simulink model "AssembledTEST1"  (R2016b)
settings: Solver=VariableStepAuto  StartTime=0.0  StopTime=60  RelTol=1e-3
values from neighbouring files (symbols this model uses):
  ail_data = [ ... (first row only)    [lookup_init.m]
  Ap = pi * (D^2)/4    (= 5.69167367599)    [constants_init.m]
  Aw = 10.0    (= 10)    [constants_init.m]
  b = 15.85    [constants_init.m]
  beta0_data = [ ... (first row only)    [lookup_init.m]
  c0 = 2.3774    [constants_init.m]
  c_i = 1.847    [constants_init.m]
  cdrag_data = [ ... (first row only)    [lookup_init.m]
  clean_wing_data = [ ... (first row only)    [lookup_init.m]
  crt = 1.6764    [constants_init.m]
  CT_data = [ ... (first row only)    [lookup_init.m]
  D = 2.692    [constants_init.m]
  D0q_10 = 0.0778    [constants_init.m]
  D0q_20 = 0.2634    [constants_init.m]
  D0q_35 = 0.7099    [constants_init.m]
  DCDi_data = [ ... (first row only)    [lookup_init.m]
  DCM0b = -0.188    [constants_init.m]
  Deh_f_on_data = [ ... (first row only)    [lookup_init.m]
  Deh_on_data = [ ... (first row only)    [lookup_init.m]
  df = 1.981    [constants_init.m]
  DOWN_0 = HP * F2M    (= 1830.0192)    [InitialiseJ31.m]    (also in Trim.m = -xtrim(12))
  Dqhq_data = [ ... (first row only)    [lookup_init.m]
  e0 = d2r(2.0)    [constants_init.m]
  e_data10 = [ ... (first row only)    [lookup_init.m]
  e_data20 = [ ... (first row only)    [lookup_init.m]
  e_data35 = [ ... (first row only)    [lookup_init.m]
  EAST_0 = 0.0    (= 0)    [InitialiseJ31.m]    (also in Trim.m = xtrim(11))
  elaw_0 = -7.50225e+2    (= -750.225)    [constants_init.m]
  elaw_1 = 8.98698    [constants_init.m]
  elaw_2 = -6.94240e-3    (= -0.0069424)    [constants_init.m]
  FLAP = 0    [InitialiseJ31.m]
  flaps_lift_data = [ ... (first row only)    [lookup_init.m]
  flaps_moment_data = [ ... (first row only)    [lookup_init.m]
  flaps_tail_data = [ ... (first row only)    [lookup_init.m]
  flaps_wing_data = [ ... (first row only)    [lookup_init.m]
  fmc_data = [ ... (first row only)    [lookup_init.m]
  fmf_data = [ ... (first row only)    [lookup_init.m]
  fmn_data = [ ... (first row only)    [lookup_init.m]
  fus_data = [ ... (first row only)    [lookup_init.m]
  gamma_t = 0.578    [constants_init.m]
  h_data10 = [ ... (first row only)    [lookup_init.m]
  h_data20 = [ ... (first row only)    [lookup_init.m]
  h_data35 = [ ... (first row only)    [lookup_init.m]
  INERTIA = [IXX,IXY,IXZ;IXY,IYY,IYZ;IXZ,IYZ,IZZ]    [InitialiseJ31.m]
  it = d2r(-2.3)    [constants_init.m]
  iw = d2r(1.33)    [constants_init.m]
  Iwn2 = 0.636    [constants_init.m]
  J_W = 1.26    [constants_init.m]
  K1_data = [ ... (first row only)    [lookup_init.m]
  k1f_data = [ ... (first row only)    [lookup_init.m]
  k_data = [ ... (first row only)    [lookup_init.m]
  L_r0_10f = -0.0096    [constants_init.m]
  L_r0_20f = -0.0180    (= -0.018)    [constants_init.m]
  L_r0_35f = -0.0245    [constants_init.m]
  l_t = 11.6205 - 5.6642    (= 5.9563)    [constants_init.m]
  ld_data = [ ... (first row only)    [lookup_init.m]
  Lt = 4.686    [constants_init.m]
  Lt_dash = 247.1 * 0.3048/12    (= 6.27634)    [constants_init.m]
  Lv_b = -0.00145    [constants_init.m]
  Lv_h = 0.0445    [constants_init.m]
  Lv_n = 0.0165    [constants_init.m]
  mac = 1.716    [constants_init.m]
  mach_ffr = 0.4158    [constants_init.m]
  mach_pow = 0.7984    [constants_init.m]
  n = 1591/60    (= 26.5166666667)    [constants_init.m]
  NORTH_0 = 0.0    (= 0)    [InitialiseJ31.m]    (also in Trim.m = xtrim(10))
  Nr_b = -0.0060    (= -0.006)    [constants_init.m]
  Nv_n = -0.0005    [constants_init.m]
  Nv_wb = -0.0719    [constants_init.m]
  P_0 = 0.0    (= 0)    [InitialiseJ31.m]    (also in Trim.m = xtrim(4))
  pdrag_data = [ ... (first row only)    [lookup_init.m]
  PHI_0 = xtrim(7)    [Trim.m]
  piAt = At * pi    (= 17.5929188601)    [constants_init.m]
  piAw = Aw * pi    (= 31.4159265359)    [constants_init.m]
  PSI_0 = xtrim(9)    [Trim.m]
  Q_0 = 0.0    (= 0)    [InitialiseJ31.m]    (also in Trim.m = xtrim(5))
  R2D = 180/pi    (= 57.2957795131)    [InitialiseJ31.m]
  R_0 = 0.0    (= 0)    [InitialiseJ31.m]    (also in Trim.m = xtrim(6))
  s_e = 0.0954    [constants_init.m]
  side_data = [ ... (first row only)    [lookup_init.m]
  sideforce_data = [ ... (first row only)    [lookup_init.m]
  Sit = 1.874    [constants_init.m]
  Sn = 0.552    [constants_init.m]
  Sref = (pi/4) * df^2    (= 3.08218592191)    [constants_init.m]
  St = 7.785    [constants_init.m]
  Sw = 25.084    [constants_init.m]
  tail_data = [ ... (first row only)    [lookup_init.m]
  THETA_0 = xtrim(8)    [Trim.m]
  U_0 = xtrim(1)    [Trim.m]
  upwash_clean = [ ... (first row only)    [lookup_init.m]
  upwash_flaps = [ ... (first row only)    [lookup_init.m]
  V_0 = xtrim(2)    [Trim.m]
  vortex_drag_factors = [ ... (first row only)    [lookup_init.m]
  W_0 = xtrim(3)    [Trim.m]
  X_ci = ((223 - 140)*0.3048/12) - Xp_dash    (= 0.09144)    [constants_init.m]
  xacf = -6.653    [constants_init.m]
  xacn = (223 - 197.3)*0.3048/12    (= 0.65278)    [constants_init.m]
  xb0 = c0 * xb0_c0    (= 0.5895952)    [constants_init.m]
  xcit = -l_t - ycit * sin(d2r(11.31)) - (0.981/4)    [constants_init.m]
  Xp_dash = 79.4  * 0.3048/12    (= 2.01676)    [constants_init.m]
  xyz_p = [140.0*0.3048/12;-107.0*0.3048/12;11.5*0.3048/12]    [constants_init.m]
  xyz_s = [140.0*0.3048/12; 107.0*0.3048/12;11.5*0.3048/12]    [constants_init.m]
  ycit = 2.306    [constants_init.m]
  Yr_b = -0.0283    [constants_init.m]
  Yv_n = -0.0458    [constants_init.m]
  Yv_wb = -0.2627    [constants_init.m]
  Z_ht = 11.5*0.3048/12 - zact    (= 1.7271)    [constants_init.m]
  zacf = -1.741    [constants_init.m]
  zacn = 11.5*0.3048/12    (= 0.2921)    [constants_init.m]
  zact = -1.435    [constants_init.m]
  zacw = 0.929 - (3.307 * tan(d2r(7)))    [constants_init.m]
  Zt_dash = 12.0  * 0.3048/12    (= 0.3048)    [constants_init.m]
undefined symbols (not defined in the file or in its folder): CG, MASS
libraries: aerolibasang x3, aerolibatmos2 x1
(part 5 of 5)

== system AssembledTEST1/Subsystem/Powerplants and Slipstream/Subsystem2/Powerplant - starboard (forces and moments about spinner) (in body axes)/Propeller - right (forces and moments about spinner) (in body axes)/upwash at spinner ==
  In4 : Inport
  In1 : Inport  Port=2
  In3 : Inport  Port=3
  In2 : Inport  Port=4
  Add : Sum
  Constant : Constant
  Get_af : Sum
  Get_an : Sum  Inputs=+++
  Get_efi : Product  RndMeth=Zero
  Get_efo : Product  RndMeth=Zero
  Get_efw : Subsystem
      mask Display:
      | port_label('output',1,'\epsilon^f_{w}','texmode','on')
      | port_label('input',1,'flap')
      | port_label('input',2,'Mach')
      | port_label('input',3,'C_L','texmode','on')
  Get_ei : Sum  Inputs=+++
  Get_en : Product  RndMeth=Zero
  Get_enf : Product  RndMeth=Zero
  Get_enw : Subsystem
      mask Display:
      | port_label('output',1,'\epsilon^n_{w}','texmode','on')
      | port_label('input',1,'flap')
      | port_label('input',2,'Mach')
      | port_label('input',3,'C_L','texmode','on')
  Get_eo : Sum  Inputs=+++
  Get_ewi : Product  RndMeth=Zero
  Get_ewi_CL : Subsystem
      mask Display:
      | port_label('output',1,'\epsilon_{wi}/C_L','texmode','on')
      | port_label('input',1,'flap')
      | port_label('input',2,'Mach')
  Get_ewo : Product  RndMeth=Zero
  Get_ewo_CL : Subsystem
      mask Display:
      | port_label('output',1,'\epsilon_{wo}/C_L','texmode','on')
      | port_label('input',1,'flap')
      | port_label('input',2,'Mach')
  Mux : Mux  Inputs=2
  Mux1 : Mux  Inputs=2
  average : Fcn  Expr=0.5*(u(1)+u(2))
  average1 : Fcn  Expr=0.5*(u(1)+u(2))
  d2r : Fcn  Expr=u(1)*pi/180
  d2r1 : Fcn  Expr=u(1)*pi/180
  efi_af : Lookup  InputValues=upwash_clean(:,1)  Table=upwash_clean(:,6)
  efo_af : Lookup  InputValues=upwash_clean(:,1)  Table=upwash_clean(:,7)
  en_an : Lookup  InputValues=upwash_clean(:,1)  Table=upwash_clean(:,9)
  enf_af : Lookup  InputValues=upwash_clean(:,1)  Table=upwash_clean(:,8)
  r2d : Fcn  Expr=u(1)*180/pi
  Out1 : Outport
  Out2 : Outport  Port=2
  wires:
  In4/1 -> r2d/1
  In3/1 -> [CL]
  In2/1 -> [Mach]
  d2r/1 -> Out1/1
  In1/1 -> Add/1
  average/1 -> d2r/1
  Get_eo/1 -> Mux/2
  Get_ei/1 -> Mux/1
  Mux/1 -> average/1
  Get_efo/1 -> Get_eo/2
  Get_en/1 -> Get_eo/3, Get_ei/3
  Get_efi/1 -> Get_ei/2
  en_an/1 -> Get_en/2
  Get_an/1 -> Get_en/1
  efo_af/1 -> Get_efo/1
  efi_af/1 -> Get_efi/1
  r2d/1 -> [alpha]
  [alpha] -> Get_an/3
  Get_enf/1 -> Get_an/1
  enf_af/1 -> Get_enf/2
  Get_af/1 -> Get_efo/2, Get_enf/1, Get_efi/2
  [Mach] -> enf_af/1
  [alpha] -> Get_af/2
  [CL] -> Get_enw/3(In2)
  [Mach] -> en_an/1, Get_enw/2(In3)
  [flap] -> Get_enw/1(In1)
  Get_enw/1(Out1) -> Get_an/2
  [CL] -> Get_efw/3(In2)
  [Mach] -> Get_efw/2(In3)
  [flap] -> Get_efw/1(In1)
  Get_efw/1(Out1) -> Get_af/1
  [Mach] -> efo_af/1, Get_ewo_CL/2(In3)
  [flap] -> Get_ewo_CL/1(In1)
  [Mach] -> efi_af/1, Get_ewi_CL/2(In3)
  [flap] -> Get_ewi_CL/1(In1)
  Constant/1 -> Add/2
  Add/1 -> [flap]
  Get_ewi/1 -> Get_ei/1
  Get_ewi_CL/1(Out1) -> Get_ewi/1, Mux1/1
  [CL] -> Get_ewi/2
  Get_ewo_CL/1(Out1) -> Get_ewo/1, Mux1/2
  Get_ewo/1 -> Get_eo/1
  [CL] -> Get_ewo/2
  Mux1/1 -> average1/1
  average1/1 -> d2r1/1
  d2r1/1 -> Out2/1

== system AssembledTEST1/Subsystem/Powerplants and Slipstream/Subsystem2/Powerplant - port (forces and moments about spinner) (in body axes)/Propeller - left (forces and moments about spinner) (in body axes)/upwash at spinner/Get_efw ==
  In1 : Inport
  In3 : Inport  Port=2
  In2 : Inport  Port=3
  Multiport Switch : MultiPortSwitch  Inputs=4
  Product : Product  RndMeth=Zero
  efw_CL_clean : Lookup  InputValues=upwash_clean(:,1)  Table=upwash_clean(:,4)
  efw_CL_flaps10 : Lookup  InputValues=upwash_flaps(:,1)  Table=upwash_flaps(:,8)
  efw_CL_flaps20 : Lookup  InputValues=upwash_flaps(:,1)  Table=upwash_flaps(:,9)
  efw_CL_flaps35 : Lookup  InputValues=upwash_flaps(:,1)  Table=upwash_flaps(:,10)
  Out1 : Outport
  wires:
  In2/1 -> Product/2
  Product/1 -> Out1/1
  In1/1 -> Multiport Switch/1
  Multiport Switch/1 -> Product/1
  In3/1 -> efw_CL_clean/1, efw_CL_flaps10/1, efw_CL_flaps20/1, efw_CL_flaps35/1
  efw_CL_clean/1 -> Multiport Switch/2
  efw_CL_flaps10/1 -> Multiport Switch/3
  efw_CL_flaps20/1 -> Multiport Switch/4
  efw_CL_flaps35/1 -> Multiport Switch/5

== system AssembledTEST1/Subsystem/Powerplants and Slipstream/Subsystem2/Powerplant - port (forces and moments about spinner) (in body axes)/Propeller - left (forces and moments about spinner) (in body axes)/upwash at spinner/Get_enw ==
  In1 : Inport
  In3 : Inport  Port=2
  In2 : Inport  Port=3
  Multiport Switch : MultiPortSwitch  Inputs=4
  Product : Product  RndMeth=Zero
  enw_CL_clean : Lookup  InputValues=upwash_clean(:,1)  Table=upwash_clean(:,5)
  enw_CL_flaps10 : Lookup  InputValues=upwash_flaps(:,1)  Table=upwash_flaps(:,11)
  enw_CL_flaps20 : Lookup  InputValues=upwash_flaps(:,1)  Table=upwash_flaps(:,12)
  enw_CL_flaps35 : Lookup  InputValues=upwash_flaps(:,1)  Table=upwash_flaps(:,13)
  Out1 : Outport
  wires:
  In2/1 -> Product/2
  Product/1 -> Out1/1
  In1/1 -> Multiport Switch/1
  Multiport Switch/1 -> Product/1
  In3/1 -> enw_CL_clean/1, enw_CL_flaps10/1, enw_CL_flaps20/1, enw_CL_flaps35/1
  enw_CL_clean/1 -> Multiport Switch/2
  enw_CL_flaps10/1 -> Multiport Switch/3
  enw_CL_flaps20/1 -> Multiport Switch/4
  enw_CL_flaps35/1 -> Multiport Switch/5

== system AssembledTEST1/Subsystem/Powerplants and Slipstream/Subsystem2/Powerplant - port (forces and moments about spinner) (in body axes)/Propeller - left (forces and moments about spinner) (in body axes)/upwash at spinner/Get_ewi_CL ==
  In1 : Inport
  In3 : Inport  Port=2
  Multiport Switch : MultiPortSwitch  Inputs=4
  ewi_CL_clean : Lookup  InputValues=upwash_clean(:,1)  Table=upwash_clean(:,2)
  ewi_CL_flaps10 : Lookup  InputValues=upwash_flaps(:,1)  Table=upwash_flaps(:,2)
  ewi_CL_flaps20 : Lookup  InputValues=upwash_flaps(:,1)  Table=upwash_flaps(:,4)
  ewi_CL_flaps35 : Lookup  InputValues=upwash_flaps(:,1)  Table=upwash_flaps(:,6)
  Out1 : Outport
  wires:
  In1/1 -> Multiport Switch/1
  In3/1 -> ewi_CL_clean/1, ewi_CL_flaps10/1, ewi_CL_flaps20/1, ewi_CL_flaps35/1
  ewi_CL_clean/1 -> Multiport Switch/2
  ewi_CL_flaps10/1 -> Multiport Switch/3
  ewi_CL_flaps20/1 -> Multiport Switch/4
  ewi_CL_flaps35/1 -> Multiport Switch/5
  Multiport Switch/1 -> Out1/1

== system AssembledTEST1/Subsystem/Powerplants and Slipstream/Subsystem2/Powerplant - port (forces and moments about spinner) (in body axes)/Propeller - left (forces and moments about spinner) (in body axes)/upwash at spinner/Get_ewo_CL ==
  In1 : Inport
  In3 : Inport  Port=2
  Multiport Switch : MultiPortSwitch  Inputs=4
  ewo_CL_clean : Lookup  InputValues=upwash_clean(:,1)  Table=upwash_clean(:,3)
  ewo_CL_flaps10 : Lookup  InputValues=upwash_flaps(:,1)  Table=upwash_flaps(:,3)
  ewo_CL_flaps20 : Lookup  InputValues=upwash_flaps(:,1)  Table=upwash_flaps(:,5)
  ewo_CL_flaps35 : Lookup  InputValues=upwash_flaps(:,1)  Table=upwash_flaps(:,7)
  Out1 : Outport
  wires:
  In1/1 -> Multiport Switch/1
  In3/1 -> ewo_CL_clean/1, ewo_CL_flaps10/1, ewo_CL_flaps20/1, ewo_CL_flaps35/1
  ewo_CL_clean/1 -> Multiport Switch/2
  ewo_CL_flaps10/1 -> Multiport Switch/3
  ewo_CL_flaps20/1 -> Multiport Switch/4
  ewo_CL_flaps35/1 -> Multiport Switch/5
  Multiport Switch/1 -> Out1/1

== system AssembledTEST1/Subsystem/Powerplants and Slipstream/Subsystem2/Powerplant - starboard (forces and moments about spinner) (in body axes)/Propeller - right (forces and moments about spinner) (in body axes)/upwash at spinner/Get_efw ==
  In1 : Inport
  In3 : Inport  Port=2
  In2 : Inport  Port=3
  Multiport Switch : MultiPortSwitch  Inputs=4
  Product : Product  RndMeth=Zero
  efw_CL_clean : Lookup  InputValues=upwash_clean(:,1)  Table=upwash_clean(:,4)
  efw_CL_flaps10 : Lookup  InputValues=upwash_flaps(:,1)  Table=upwash_flaps(:,8)
  efw_CL_flaps20 : Lookup  InputValues=upwash_flaps(:,1)  Table=upwash_flaps(:,9)
  efw_CL_flaps35 : Lookup  InputValues=upwash_flaps(:,1)  Table=upwash_flaps(:,10)
  Out1 : Outport
  wires:
  In2/1 -> Product/2
  Product/1 -> Out1/1
  In1/1 -> Multiport Switch/1
  Multiport Switch/1 -> Product/1
  In3/1 -> efw_CL_clean/1, efw_CL_flaps10/1, efw_CL_flaps20/1, efw_CL_flaps35/1
  efw_CL_clean/1 -> Multiport Switch/2
  efw_CL_flaps10/1 -> Multiport Switch/3
  efw_CL_flaps20/1 -> Multiport Switch/4
  efw_CL_flaps35/1 -> Multiport Switch/5

== system AssembledTEST1/Subsystem/Powerplants and Slipstream/Subsystem2/Powerplant - starboard (forces and moments about spinner) (in body axes)/Propeller - right (forces and moments about spinner) (in body axes)/upwash at spinner/Get_enw ==
  In1 : Inport
  In3 : Inport  Port=2
  In2 : Inport  Port=3
  Multiport Switch : MultiPortSwitch  Inputs=4
  Product : Product  RndMeth=Zero
  enw_CL_clean : Lookup  InputValues=upwash_clean(:,1)  Table=upwash_clean(:,5)
  enw_CL_flaps10 : Lookup  InputValues=upwash_flaps(:,1)  Table=upwash_flaps(:,11)
  enw_CL_flaps20 : Lookup  InputValues=upwash_flaps(:,1)  Table=upwash_flaps(:,12)
  enw_CL_flaps35 : Lookup  InputValues=upwash_flaps(:,1)  Table=upwash_flaps(:,13)
  Out1 : Outport
  wires:
  In2/1 -> Product/2
  Product/1 -> Out1/1
  In1/1 -> Multiport Switch/1
  Multiport Switch/1 -> Product/1
  In3/1 -> enw_CL_clean/1, enw_CL_flaps10/1, enw_CL_flaps20/1, enw_CL_flaps35/1
  enw_CL_clean/1 -> Multiport Switch/2
  enw_CL_flaps10/1 -> Multiport Switch/3
  enw_CL_flaps20/1 -> Multiport Switch/4
  enw_CL_flaps35/1 -> Multiport Switch/5

== system AssembledTEST1/Subsystem/Powerplants and Slipstream/Subsystem2/Powerplant - starboard (forces and moments about spinner) (in body axes)/Propeller - right (forces and moments about spinner) (in body axes)/upwash at spinner/Get_ewi_CL ==
  In1 : Inport
  In3 : Inport  Port=2
  Multiport Switch : MultiPortSwitch  Inputs=4
  ewi_CL_clean : Lookup  InputValues=upwash_clean(:,1)  Table=upwash_clean(:,2)
  ewi_CL_flaps10 : Lookup  InputValues=upwash_flaps(:,1)  Table=upwash_flaps(:,2)
  ewi_CL_flaps20 : Lookup  InputValues=upwash_flaps(:,1)  Table=upwash_flaps(:,4)
  ewi_CL_flaps35 : Lookup  InputValues=upwash_flaps(:,1)  Table=upwash_flaps(:,6)
  Out1 : Outport
  wires:
  In1/1 -> Multiport Switch/1
  In3/1 -> ewi_CL_clean/1, ewi_CL_flaps10/1, ewi_CL_flaps20/1, ewi_CL_flaps35/1
  ewi_CL_clean/1 -> Multiport Switch/2
  ewi_CL_flaps10/1 -> Multiport Switch/3
  ewi_CL_flaps20/1 -> Multiport Switch/4
  ewi_CL_flaps35/1 -> Multiport Switch/5
  Multiport Switch/1 -> Out1/1

== system AssembledTEST1/Subsystem/Powerplants and Slipstream/Subsystem2/Powerplant - starboard (forces and moments about spinner) (in body axes)/Propeller - right (forces and moments about spinner) (in body axes)/upwash at spinner/Get_ewo_CL ==
  In1 : Inport
  In3 : Inport  Port=2
  Multiport Switch : MultiPortSwitch  Inputs=4
  ewo_CL_clean : Lookup  InputValues=upwash_clean(:,1)  Table=upwash_clean(:,3)
  ewo_CL_flaps10 : Lookup  InputValues=upwash_flaps(:,1)  Table=upwash_flaps(:,3)
  ewo_CL_flaps20 : Lookup  InputValues=upwash_flaps(:,1)  Table=upwash_flaps(:,5)
  ewo_CL_flaps35 : Lookup  InputValues=upwash_flaps(:,1)  Table=upwash_flaps(:,7)
  Out1 : Outport
  wires:
  In1/1 -> Multiport Switch/1
  In3/1 -> ewo_CL_clean/1, ewo_CL_flaps10/1, ewo_CL_flaps20/1, ewo_CL_flaps35/1
  ewo_CL_clean/1 -> Multiport Switch/2
  ewo_CL_flaps10/1 -> Multiport Switch/3
  ewo_CL_flaps20/1 -> Multiport Switch/4
  ewo_CL_flaps35/1 -> Multiport Switch/5
  Multiport Switch/1 -> Out1/1

== matlab function AssembledTEST1/Equations of Motion/Navigation_equations/DCM_matrix ==
  data: EUL input; T output
function T  = DCM(EUL)

%Euler Angles
Phi   = EUL(1);
Theta = EUL(2);
Psi   = EUL(3);

%% Cosine Matrix

T = zeros (3,3);

T(1,1) = cos(Theta)*cos(Psi);
T(1,2) = cos(Theta)*sin(Psi);
T(1,3) = -sin(Theta);

T(2,1) = -cos(Phi)*sin(Psi) + sin(Phi)*sin(Theta)*cos(Psi);
T(2,2) = cos(Phi)*cos(Psi) +sin(Phi)*sin(Theta)*sin(Psi);
T(2,3) = sin(Phi)*cos(Theta);

T(3,1) = sin(Phi)*sin(Psi) + cos(Phi)*sin(Theta)*cos(Psi);
T(3,2) = -sin(Phi)*cos(Psi)+ cos(Phi)*sin(Theta)*sin(Psi);
T(3,3) = cos(Phi)*cos(Theta);
end

== matlab function AssembledTEST1/Equations of Motion/EoMs ==
  data: Forces input; Vdot output; Moments input; velocity input; omega input; omegadot output; MASS input; INERTIA input; CG input
function [Vdot,omegadot]= Equations_of_Motion(Forces,Moments,velocity,omega,MASS,INERTIA,CG)
%Variable definition
m=MASS;
dx=CG(1);
dy=CG(2);
dz=CG(3);
I=INERTIA;
Ixx=I(1,1);
Iyy=I(2,2);
Izz=I(3,3);
Ixz=I(1,3);


U=velocity(1);
V=velocity(2);
W=velocity(3);

P=omega(1);
Q=omega(2);
R=omega(3);


X=Forces(1);
Y=Forces(2);
Z=Forces(3);

L=Moments(1);
M=Moments(2);
N=Moments(3);

% Motion's Matrix composition


massProperties=[
        m       0       0       0       m*dz   -m*dy;
        0       m       0      -m*dz    0       m*dx;
        0       0       m       m*dy   -m*dx    0   ;
        0      -m*dz    m*dy    Ixx     0      -Ixz ;
        m*dz    0      -m*dx    0       Iyy     0   ;
       -m*dy    m*dx    0      -Ixz     0       Izz  ];
   
dynamicProperties=[
        X+m*R*V-m*Q*W+m*dx*(Q^2+R^2)-m*dy*P*Q-m*dz*P*R;
        Y-m*R*U+m*P*W-m*dx*P*Q+m*dy*(P^2+R^2)-m*dz*Q*R;
        Z+m*Q*U-m*P*V-m*dx*P*R+m*dy*Q*R+m*dz*(P^2+Q^2);
        L-Q*R*(Izz-Iyy)+P*Q*Ixz-(P*V-Q*U)*m*dy+(R*U-P*W)*m*dz;
        M-P*R*(Ixx-Izz)-(P^2-R^2)*Ixz-(Q*U-P*V)*m*dx-(Q*W-R*V)*m*dz;
        N-P*Q*(Iyy-Ixx)-Q*R*Ixz-(R*U-P*W)*m*dx+(Q*W-R*V)*m*dy];
 
% Motion output
    
motion=massProperties\dynamicProperties;  


Vdot        =motion(1:3);
omegadot    =motion(4:6);

%Problemes:
%dx in angular

end

== matlab function AssembledTEST1/Subsystem/Lateral//Directional Aerodynamics/getYLN/Embedded MATLAB Function ==
  data: sigma input; Lv_b input; alpha input; Yv output; Yv_f input; Yv_v input; Y_rud input; Lv_di input; Lv_w_CL input; Np_w_CL input; Yp_w_CL input; a1_wb input; Lp_w input; CLw input; CLb input; Yv_wb input; Yv_n input; Yr_b input; Lv_n input; Lv_h input; Nv_wb input; Nv_n input; Nr_b input; J_W input; Yp output; Yr output; Y_zeta output; Lv output; Lp output; Lr output; L_zeta output; Nv output; Lr_0_f input; Lr_Lr0 input; Np output; Nr output; N_zeta output; b input; CD0w input; DelCDi_flap input; DelCD0_flap input
function [Yv,Yp,Yr,Y_zeta,Lv,Lp,Lr,L_zeta,Nv,Np,Nr,N_zeta] = Get_YLNderivs(sigma,Lv_b,alpha,Yv_f,Yv_v,Y_rud,Lv_di,Lv_w_CL,Np_w_CL,Yp_w_CL,a1_wb,Lp_w,CLw,CLb,Yv_wb,Yv_n,Yr_b,Lv_n,Lv_h,Nv_wb,Nv_n,Nr_b,J_W,Lr_0_f,Lr_Lr0,b,CD0w,DelCDi_flap,DelCD0_flap)

%CL_w,Dv_wing,D0_wing,p,q,r,Mach,V,alpha,beta,qbar,Aileron_L,Aileron_R,Rudder,Flap,wdot,xcg)

%   This function determines the side force, rolling momement and yawing
%   moment at the specified dynamic pressure.
%   Uses the methods given in ESDU 79006, 82010, 87008, 81013, 80033,
%   80034, 00025, 73006, A.06.01.03, 83006, 92029, 72021, 83026, 82017,
%   88029
%
%   Author: A Cooke Date:   1 Jun 05, modified 12 Jan 06, 16 Jun 06
%   Converted to embedded MatLab Function 31 Oct 07

% Yv_f  = sideforce derivative for fin 
Lv_f    =  (Yv_f/b) * (1.571 * cos(alpha) - 6.339 * sin(alpha));   % rolling moment derivative for fin
Nv_f    = -(Yv_f/b) * (6.339 * cos(alpha) + 1.571 * sin(alpha));   % yawing moment derivative for fin

% Yv_v  = sideforce derivative for ventral fin 
Lv_v    = -(Yv_v/b) * (0.524 * cos(alpha) + 6.335 * sin(alpha));   % rolling moment derivative for ventral fin 
Nv_v    = -(Yv_v/b) * (6.335 * cos(alpha) - 0.524 * sin(alpha));   % yawing moment derivative for ventral fin 

Yp_f    = -1.377 * (0.060 * cos(alpha) - 0.444 * sin(alpha) - 0.18 - sigma);  % sideforce derivative for fin
Lp_f    =  (Yp_f/b) * (0.946 * cos(alpha) - 7.042 * sin(alpha));     % rolling moment derivative for fin
Np_f    = -(Yp_f/b) * (7.042 * cos(alpha) + 0.946 * sin(alpha));     % yawing moment derivative for fin

Yr_f    = -(Yv_f/(b * J_W)) * (6.339 * cos(alpha) + 1.571 * sin(alpha));% sideforce derivative for fin
Lr_f    =  (Yr_f/b) * (1.571 * cos(alpha) - 6.339 * sin(alpha));        % rolling moment derivative for fin
Nr_f    = -(Yr_f/b) * (6.339 * cos(alpha) + 1.571 * sin(alpha));        % yawing moment derivative for fin

% Y_zeta  = sideforce derivative for rudder 
Y_zeta  = Y_rud * cos(32.3 * pi/180);      % conversion as rudder deflection normal to hinge line
L_zeta  =  (Y_zeta/b) * (1.498 * cos(alpha) - 6.833 * sin(alpha));  % rolling moment derivative for rudder
N_zeta  = -(Y_zeta/b) * (6.833 * cos(alpha) + 1.498 * sin(alpha));  % yawing moment derivative for rudder

DelCL_flap = CLw - CLb;   % determine increment in lift due to flap deployment        

Lv_w    = Lv_w_CL * CLb;                                 % rolling moment derivative from planform 
Yp_w    = Yp_w_CL * CLb;                                 % sideforce derivative from planform 
Np_w    = (Np_w_CL + 0.000038 * a1_wb) * CLb;            % yawing moment derivative from planform

Lv_flap = 0.0322 * DelCL_flap;                                 % rolling moment derivative from flap deployment 
Yv_flap = -DelCDi_flap + (0.045 * Yv_f + 0.003) * DelCL_flap;  % sideforce derivative from flap deployment
Nv_flap = 0.196 * DelCDi_flap + 0.045 * Nv_f * DelCL_flap;     % yawing moment derivative from flap deployment

Yp_di  =  0.3924 * Lp_w;                                % sideforce derivative from dihedral
Lp_di  = -0.0466 * Lp_w;                                % rolling moment derivative from dihedral
Np_di  =  0.0019 * Lp_w;                                % yawing moment derivative from dihedral

Nr_w = -0.1238 * (CD0w + 0.305 * DelCD0_flap) - 0.0053 * CLw^2; % yawing moment derivative from wing/flap

Lr_w    = (0.109 * CLw - 0.0037 + Lr_0_f) * Lr_Lr0;     % rolling moment derivative from wing/flap

% summation of derivatives

Yv      = Yv_wb + Yv_n + Yv_f + Yv_flap + Yv_v;
Yp      = Yp_w + Yp_di + Yp_f;
Yr      = Yr_b + Yr_f;

% Y_fin_w   = (qbar/V) * Sw * (Yv_f * v +  b * (Yp_f * p + Yr_f * r)) + Yrud * Rudder;    % total fin sideforce wind axes

Lv      = Lv_n + Lv_f + Lv_di + Lv_w + Lv_b + Lv_h + Lv_flap + Lv_v;
Lp      = Lp_w + Lp_di + Lp_f;
Lr      = Lr_w + Lr_f;

Nv      = Nv_wb + Nv_n + Nv_f + Nv_flap + Nv_v;
Np      = Np_w + Np_di + Np_f;
Nr      = Nr_w + Nr_b + Nr_f;

== matlab function AssembledTEST1/Subsystem/Lateral//Directional Aerodynamics/getYLN/Embedded MATLAB Function1 ==
  data: V input; alpha input; beta input; qbar input; Sw input; b input; Yv input; Y output; Yp input; Yr input; Yzeta input; Lv input; Lp input; Lr input; Lzeta input; Nv input; Np input; Nr input; Nzeta input; p input; r input; Rudder input; Nxi input; Lxi input; L output; N output
function [Y,L,N] = Get_YLN(V,alpha,beta,qbar,Sw,b,Yv,Yp,Yr,Yzeta,Lv,Lp,Lr,Lzeta,Nv,Np,Nr,Nzeta,p,r,Rudder,Nxi,Lxi)
% This function determines the lateral and driectional forces and moments

% written by A Cooke : 1 Nov 07

v       = V * sin(beta);

%---------- denormalising derivatives --------

Yv      = (qbar/V) * Sw * Yv;
Yp      = (qbar/V) * Sw * b * Yp;
Yr      = (qbar/V) * Sw * b * Yr;
Yzeta   = qbar * Sw * Yzeta;

Lv      = (qbar/V) * Sw * b * Lv;
Lp      = (qbar/V) * Sw * b^2 * Lp;
Lr      = (qbar/V) * Sw * b^2 * Lr;
Lrud    = qbar * Sw * b * Lzeta;
L_ail   = qbar * Sw * b * Lxi;                  % moment NOT derivative

Nv      = (qbar/V) * Sw * b * Nv;
Np      = (qbar/V) * Sw * b^2 * Np;
Nr      = (qbar/V) * Sw * b^2 * Nr;
Nrud    = qbar * Sw * b * Nzeta;
N_ail   = qbar * Sw * b * Nxi;                  % moment NOT derivative  


%---------- conversion to body axes ----------

Yv_by    = Yv;
Yrud_by  = Yzeta;
Yp_by    = Yp * cos(alpha) - Yr * sin(alpha);
Yr_by    = Yr * cos(alpha) + Yp * sin(alpha);

Y         = Yv_by * v + Yp_by * p + Yr_by * r + Yrud_by * Rudder; % total sideforce

Lv_by    = Lv * cos(alpha) - Nv * sin(alpha);
Lrud_by  = Lrud * cos(alpha) - Nrud * sin(alpha);
L_ail_by = L_ail * cos(alpha) - N_ail * sin(alpha);
Lp_by    = Lp * cos(alpha)^2 + Nr * sin(alpha)^2 - (Lr + Np) * sin(alpha) * cos(alpha);
Lr_by    = Lr * cos(alpha)^2 - Np * sin(alpha)^2 - (Lp - Nr) * sin(alpha) * cos(alpha);

Nv_by    = Nv * cos(alpha) + Lv * sin(alpha);
Nrud_by  = Nrud * cos(alpha) + Lrud * sin(alpha);
N_ail_by = N_ail * cos(alpha) + L_ail * sin(alpha);
Np_by    = Np * cos(alpha)^2 - Lr * sin(alpha)^2 + (Lp - Nr) * sin(alpha) * cos(alpha);
Nr_by    = Nr * cos(alpha)^2 + Lp * sin(alpha)^2 + (Lr + Np) * sin(alpha) * cos(alpha);

L       = Lv_by * v + Lr_by * r + Lp_by * p + Lrud_by * Rudder + L_ail_by; % total rolling moment
N       = Nv_by * v + Nr_by * r + Np_by * p + Nrud_by * Rudder + N_ail_by; % total yawing moment

== matlab function AssembledTEST1/Subsystem/Longitudinal Aerodynamics/Get Drag/Embedded MATLAB Function ==
  data: Sw input; qh_q output; Aw input; mac input; Lt input; gamma_t input; alpha_w input; Dqw input; CLw input
function qh_q = Get_qhq(Sw,Aw,mac,Lt,gamma_t,alpha_w,Dqw,CLw)

% this function determines the power-off dynamic pressure at
% the tailplane using NASA TN D-6800

% written by A Cooke - 12 Sep 07

CDw = Dqw/Sw;
eh  = (1.62 * CLw)/(pi * Aw);   % downwash in plane of symmetry
mu  = gamma_t + eh - alpha_w;

X = Lt * cos(mu);
Z = Lt * sin(mu);

delZ_mac = 0.68 * sqrt(CDw * ((X/mac) + 0.15));
delZ     = delZ_mac * mac;

delq_q0  = (2.42 * sqrt(CDw))/((X/mac) + 0.3);

if (Z/delZ) > 1.0
    delq_q = 0.0;
else
    delq_q = delq_q0 * (cos((pi/2)*(Z/delZ)))^2;
end

qh_q = 1 - delq_q;

== matlab function AssembledTEST1/Subsystem/Powerplants and Slipstream/Subsystem2/Powerplant - port (forces and moments about spinner) (in body axes)/Embedded MATLAB Function ==
  data: Xp_dash input; Ai output; Zt_dash input; Dp input; c_i input; alpha_b input; upwash input; downwash_p input; Si output
function [Ai,Si] = GetARimmersed(Xp_dash,Zt_dash,Dp,c_i,alpha_b,upwash,downwash_p)

% This fuction detemines the aspect ratio of the portion of the wing
% immersed in the propeller slipstream. Taken from NASA TN D-6800

% written by A Cooke 3 Aug 07

Zs_dash = Zt_dash + Xp_dash * tan(alpha_b + upwash - downwash_p);
b_i     = 2 * sqrt((Dp/2)^2 + Zs_dash^2);
Ai      = b_i/c_i;
Si      = b_i*c_i;

== matlab function AssembledTEST1/Subsystem/Powerplants and Slipstream/Subsystem2/Powerplant - port (forces and moments about spinner) (in body axes)/Embedded MATLAB Function1 ==
  data: deuda input; CLw input; Sw input; TC input; K1 input; Si input; ep input; DCLw_slip output; D0qw_slip output; D0qw input; a1 input
function [DCLw_slip,D0qw_slip] = Get_CLD0qw_slip(deuda,CLw,Sw,TC,K1,Si,ep,D0qw,a1)

% Thus function determines the contribution to wing CL and D0/q made by
% the propeller slipstream using NASA TN D-6800

% written by A Cooke: 14 Aug 07, modified 24 Jan 08

delqbarw_qbar = TC * 8/pi;
delalpha_si   = -ep/(1 - deuda);

D0qw_slip = D0qw * (Si/Sw) * delqbarw_qbar;
DCLw_slip = CLw * (Si/Sw) * K1 * delqbarw_qbar;
DCLw_slip = DCLw_slip + ((Si/Sw) * a1 * delalpha_si * (1 + delqbarw_qbar));

== matlab function AssembledTEST1/Subsystem/Powerplants and Slipstream/Subsystem2/Embedded MATLAB Function ==
  data: X input; L output; Y input; Z input; xyz input; M output; N output
function [L,M,N] = getLMN(X,Y,Z,xyz)
% This block converts propeller forces into moments
% about the Body Axes Centre

x = xyz(1);
y = xyz(2);
z = xyz(3);
L = Z*y - Y*z;
M = X*z - Z*x;
N = Y*x - X*y;

== matlab function AssembledTEST1/Subsystem/Powerplants and Slipstream/Subsystem2/Embedded MATLAB Function1 ==
  data: X input; L output; Y input; Z input; xyz input; M output; N output
function [L,M,N] = getLMN(X,Y,Z,xyz)
% This block converts propeller forces into moments
% about the Body Axes Centre

x = xyz(1);
y = xyz(2);
z = xyz(3);
L = Z*y - Y*z;
M = X*z - Z*x;
N = Y*x - X*y;

== matlab function AssembledTEST1/Subsystem/Powerplants and Slipstream/Subsystem2/Embedded MATLAB Function2 ==
  data: Cm0w input; Cm0i output; Sw input; mac input; b input; S_ip input; S_is input; c_i input
function Cm0i = getCm0i(Cm0w,Sw,mac,b,S_ip,S_is,c_i)

% This function determines the zero lift pitching moment of the 
% basic wing for that portion not influenced by the propeller slipstreams

% written by A Cooke : 9 Oct 07

b_ip = S_ip/c_i;
b_is = S_is/c_i;

Cm0i = Cm0w*(1 - (((Sw - S_ip - S_is)^2)/(Sw*mac*(b - b_ip - b_is))));

== matlab function AssembledTEST1/Subsystem/Powerplants and Slipstream/Subsystem2/Embedded MATLAB Function3 ==
  data: X output; Lift input; Drag input; Pitch input; alpha input; Y output; Z output; L output; M output; N output; x input; z input; xyz input
function [X,Y,Z,L,M,N]  = getSlipFM(Lift,Drag,Pitch,alpha,x,z,xyz)
% This function converts the increments in lift, drag
% and pitching moment for the wing caused by the 
% propellor slipstream into forces and moments at 
% the body axes centre

% written by A Cooke : 16 Oct 07

x = xyz(1) - x;
y = xyz(2);
z = xyz(3) + z;
X =  Lift * sin(alpha) - Drag * cos(alpha);
Y = 0.0;
Z = -Lift * cos(alpha) - Drag * sin(alpha);
L = Z*y - Y*z;
M = X*z - Z*x + Pitch;
N = Y*x - X*y;

== matlab function AssembledTEST1/Subsystem/Powerplants and Slipstream/Subsystem2/Embedded MATLAB Function4 ==
  data: X output; Lift input; Drag input; Pitch input; alpha input; Y output; Z output; L output; M output; N output; x input; z input; xyz input
function [X,Y,Z,L,M,N]  = getSlipFM(Lift,Drag,Pitch,alpha,x,z,xyz)
% This function converts the increments in lift, drag
% and pitching moment for the wing caused by the 
% propellor slipstream into forces and moments at 
% the body axes centre

% written by A Cooke : 16 Oct 07

x = xyz(1) - x;
y = xyz(2);
z = xyz(3) + z;
X =  Lift * sin(alpha) - Drag * cos(alpha);
Y = 0.0;
Z = -Lift * cos(alpha) - Drag * sin(alpha);
L = Z*y - Y*z;
M = X*z - Z*x + Pitch;
N = Y*x - X*y;

== matlab function AssembledTEST1/Subsystem/Powerplants and Slipstream/Subsystem2/Get_delDi/GetDelCDi ==
  data: KDi input; alpha input; delDi output; bar_e_ep input; Xp input; Zp input; CLw input; deu_dap input; qbar input; Sw input; Aw input; b input; CDiw input; D input
function delDi = getDelDi(KDi,alpha,bar_e_ep,Xp,Zp,CLw,deu_dap,qbar,Sw,Aw,b,CDiw,D)
% This block estimates DelCDi using method from NASA TN D-6800
% written by: A Cooke -  22 Oct 07

CL_ddash = CLw + ((Xp * sin(alpha) - Zp * cos(alpha))/(qbar * Sw));
ebar     = bar_e_ep * deu_dap * alpha;
factor1  = ((CLw/CL_ddash)^2)*(1 + (pi* Aw *ebar)/CLw);
factor2  = ((b/D) * ((Xp * sin(alpha) - Zp * cos(alpha))/(qbar * Sw * CL_ddash)))^2;
delCDi   = CDiw * (factor1 + (KDi * factor2) - 1);
delDi    = delCDi * Sw * qbar;

== matlab function AssembledTEST1/Subsystem/Powerplants and Slipstream/Subsystem2/Get_delDi1/GetDelCDi ==
  data: KDi input; alpha input; delDi output; bar_e_ep input; Xp input; Zp input; CLw input; deu_dap input; qbar input; Sw input; Aw input; b input; CDiw input; D input
function delDi = getDelDi(KDi,alpha,bar_e_ep,Xp,Zp,CLw,deu_dap,qbar,Sw,Aw,b,CDiw,D)
% This block estimates DelCDi using method from NASA TN D-6800
% written by: A Cooke -  22 Oct 07

CL_ddash = CLw + ((Xp * sin(alpha) - Zp * cos(alpha))/(qbar * Sw));
ebar     = bar_e_ep * deu_dap * alpha;
factor1  = ((CLw/CL_ddash)^2)*(1 + (pi* Aw *ebar)/CLw);
factor2  = ((b/D) * ((Xp * sin(alpha) - Zp * cos(alpha))/(qbar * Sw * CL_ddash)))^2;
delCDi   = CDiw * (factor1 + (KDi * factor2) - 1);
delDi    = delCDi * Sw * qbar;

== matlab function AssembledTEST1/Subsystem/Powerplants and Slipstream/Subsystem2/Embedded MATLAB Function5 ==
  data: Cm0i input; Sw input; S_i input; mac input; c_i input; DelCM output; TC input; DelCL input; xw input
function DelCM = getDelCm(Cm0i,Sw,S_i,mac,c_i,TC,DelCL,xw)

% This function determines the pitching moment increment 
% caused by the propeller slipstream

% written by A Cooke : 23 Oct 07

Del_qw_qbar = TC * 8/pi;

DelCM0_qw = Del_qw_qbar * (S_i/Sw) * (c_i/mac) * Cm0i;
DelCM_wL  = -DelCL * (xw/mac);
DelCM = DelCM0_qw + DelCM_wL;

== matlab function AssembledTEST1/Subsystem/Powerplants and Slipstream/Subsystem2/Powerplant - port (forces and moments about spinner) (in body axes)/Get_Del_qhq/Embedded MATLAB Function ==
  data: Flap input; Del_eh_power output; Deh_power input; Deh_power_flap input
function Del_eh_power = Get_Del_eh(Flap,Deh_power,Deh_power_flap)

if Flap > 0
   Del_eh_power = Deh_power_flap;
else
   Del_eh_power = Deh_power;
end

== matlab function AssembledTEST1/Subsystem/Powerplants and Slipstream/Subsystem2/Powerplant - port (forces and moments about spinner) (in body axes)/Get_Del_qhq/Embedded MATLAB Function1 ==
  data: ep input; DelMp_q output; eu input; TC input; Iwn2 input
function DelMp_q = getDelMp(ep,eu,TC,Iwn2)
% This block determines the change in free moments for the
% nacelle due to slipstream effects, see NASA TN D-6800

% Author: A Cooke - 26 Oct 07

Del_qw_q = TC * 8/pi;
DelMp_q = (180/pi)*(eu - ep)*(1 + Del_qw_q)*Iwn2/36.5;

== matlab function AssembledTEST1/Subsystem/Powerplants and Slipstream/Subsystem2/Embedded MATLAB Function6 ==
  data: Cm0i input; Sw input; S_i input; mac input; c_i input; DelCM output; TC input; DelCL input; xw input
function DelCM = getDelCm(Cm0i,Sw,S_i,mac,c_i,TC,DelCL,xw)

% This function determines the pitching moment increment 
% caused by the propeller slipstream

% written by A Cooke : 23 Oct 07

Del_qw_qbar = TC * 8/pi;

DelCM0_qw = Del_qw_qbar * (S_i/Sw) * (c_i/mac) * Cm0i;
DelCM_wL  = -DelCL * (xw/mac);
DelCM = DelCM0_qw + DelCM_wL;

== matlab function AssembledTEST1/Subsystem/Powerplants and Slipstream/Subsystem2/Embedded MATLAB Function7 ==
  data: Lift input; X output; Drag input; alpha input; x input; y input; z input; Y output; Z output; L output; M output; N output
function [X,Y,Z,L,M,N]  = getSlipFMt(Lift,Drag,alpha,x,y,z)
% This function converts the increments in lift, drag
% and pitching moment for the tail caused by the 
% propellor slipstream into forces and moments at 
% the body axes centre

% written by A Cooke : 22 Nov 07

X =  Lift * sin(alpha) - Drag * cos(alpha);
Y = 0.0;
Z = -Lift * cos(alpha) - Drag * sin(alpha);
L = Z*y - Y*z;
M = X*z - Z*x;
N = Y*x - X*y;

== matlab function AssembledTEST1/Subsystem/Powerplants and Slipstream/Subsystem2/Embedded MATLAB Function8 ==
  data: Lift input; X output; Drag input; alpha input; x input; y input; z input; Y output; Z output; L output; M output; N output
function [X,Y,Z,L,M,N]  = getSlipFMt(Lift,Drag,alpha,x,y,z)
% This function converts the increments in lift, drag
% and pitching moment for the tail caused by the 
% propellor slipstream into forces and moments at 
% the body axes centre

% written by A Cooke : 22 Nov 07

X =  Lift * sin(alpha) - Drag * cos(alpha);
Y = 0.0;
Z = -Lift * cos(alpha) - Drag * sin(alpha);
L = Z*y - Y*z;
M = X*z - Z*x;
N = Y*x - X*y;

== matlab function AssembledTEST1/Subsystem/Powerplants and Slipstream/Subsystem2/Powerplant - port (forces and moments about spinner) (in body axes)/Propeller - left (forces and moments about spinner) (in body axes)/Embedded MATLAB Function ==
  data: CT input; beta0 input; sigma_e input; CZ_alpha output; CN_alpha output; J input
function [CZ_alpha,CN_alpha] = PropDevs(CT,beta0,sigma_e,J)

% This function determines the propeller derivatives
% at the specified Power Coefficient and Advance Ratio
%
% Author: A Cooke Date: 7 Jun 06, modified 26 Oct 06

Tc = CT * 8/(pi * J^2);
kb = tan(d2r(beta0 - 5))/(sigma_e * cos(d2r(beta0 - 5)));
CZ_alpha = -((4.25 * sigma_e)/(1 + 2 * sigma_e)) * sin(d2r(beta0 + 3)) * (1 + ((3 * Tc/8)/sqrt(1 + (2*Tc/3))));
CZ_alpha = CZ_alpha * (CT/Tc);
CN_CZ    = -(0.321/(sigma_e + tan(d2r(beta0 + 5)))) * (1 + ((Tc * kb/3)/(1 + (3 * Tc * sqrt(kb)/4))));
CN_alpha = CN_CZ * CZ_alpha;

function rad = d2r(deg)

%   This function converts degrees to radians
%
%   Author: A Cooke Date: 5 May 2004

rad = deg * pi/180;

== matlab function AssembledTEST1/Subsystem/Powerplants and Slipstream/Subsystem2/Powerplant - starboard (forces and moments about spinner) (in body axes)/Embedded MATLAB Function ==
  data: Xp_dash input; Ai output; Zt_dash input; Dp input; c_i input; alpha_b input; upwash input; downwash_p input; Si output
function [Ai,Si] = GetARimmersed(Xp_dash,Zt_dash,Dp,c_i,alpha_b,upwash,downwash_p)

% This fuction detemines the aspect ratio of the portion of the wing
% immersed in the propeller slipstream. Taken from NASA TN D-6800

% written by A Cooke 3 Aug 07

Zs_dash = Zt_dash + Xp_dash * tan(alpha_b + upwash - downwash_p);
b_i     = 2 * sqrt((Dp/2)^2 + Zs_dash^2);
Ai      = b_i/c_i;
Si      = b_i*c_i;

== matlab function AssembledTEST1/Subsystem/Powerplants and Slipstream/Subsystem2/Powerplant - starboard (forces and moments about spinner) (in body axes)/Embedded MATLAB Function1 ==
  data: deuda input; CLw input; Sw input; TC input; K1 input; Si input; ep input; DCLw_slip output; D0qw_slip output; D0qw input; a1 input
function [DCLw_slip,D0qw_slip] = Get_CLD0qw_slip(deuda,CLw,Sw,TC,K1,Si,ep,D0qw,a1)

% Thus function determines the contribution to wing CL and D0/q made by
% the propeller slipstream using NASA TN D-6800

% written by A Cooke: 14 Aug 07, modified 24 Jan 08

delqbarw_qbar = TC * 8/pi;
delalpha_si   = -ep/(1 - deuda);

D0qw_slip = D0qw * (Si/Sw) * delqbarw_qbar;
DCLw_slip = CLw * (Si/Sw) * K1 * delqbarw_qbar;
DCLw_slip = DCLw_slip + ((Si/Sw) * a1 * delalpha_si * (1 + delqbarw_qbar));

== matlab function AssembledTEST1/Subsystem/Powerplants and Slipstream/Subsystem2/Powerplant - starboard (forces and moments about spinner) (in body axes)/Get_Del_qhq/Embedded MATLAB Function ==
  data: Flap input; Del_eh_power output; Deh_power input; Deh_power_flap input
function Del_eh_power = Get_Del_eh(Flap,Deh_power,Deh_power_flap)

if Flap > 0
   Del_eh_power = Deh_power_flap;
else
   Del_eh_power = Deh_power;
end

== matlab function AssembledTEST1/Subsystem/Lateral//Directional Aerodynamics/getYLN/get_n_xi/Embedded MATLAB Function ==
  data: xi_s input; C_np output; xi_p input
function C_np = get_Cnp(xi_s,xi_p)
% This block outputs the yaw moment coefficient due to the profile drag casued by
% aileron deflection, uses ESDU 88029

% written by A Cooke: 10 Jan 08

if xi_s == 0.0
    if xi_p == 0.0
        C_np = 0.0;
    else
        C_np = 0.0119 * (0.0 - (1 - 0.0665 * (1 + (abs(xi_p)/xi_p)))*(0.0897 - xi_p)^2);
    end
elseif xi_p == 0.0
    C_np    = 0.0119 * ((1 - 0.0665 * (1 - (abs(xi_s)/xi_s)))*(0.0897 + xi_s)^2 - 0.0);
else
C_np    = 0.0119 * ((1 - 0.0665 * (1 - (abs(xi_s)/xi_s)))*(0.0897 + xi_s)^2 - (1 - 0.0665 * (1 + (abs(xi_p)/xi_p)))*(0.0897 - xi_p)^2);
end

== matlab function AssembledTEST1/Subsystem/Longitudinal Aerodynamics/Get Fuselage XZM/Embedded MATLAB Function ==
  data: Dq input; Mq input; CN input; CM input; X output; qbar input; q input; Sref input; df input; Sw input; mac input; CM0 input; Z output; M output
function [X,Z,M] = Get_XZMfus(Dq,Mq,CN,CM,qbar,q,Sref,df,Sw,mac,CM0)

% This function determines the fuselage contribution to the
% X force, Z force and M moment.

% written by A Cooke, 16 Jan 10

X  = -qbar * Dq;
Z  = -qbar * Sref * CN;
M  = -qbar * Sref * CM * df;
M0 = mac * qbar * Sw * CM0;
M  = M + M0 + (Mq * q * qbar * Sw * mac^2);

return

== matlab function AssembledTEST1/Subsystem/Lateral//Directional Aerodynamics/getYLN/slipstream effects ==
  data: b input; Xp_dash input; xp input; yp input; Xp input; Yv_ns output; Lv_s output; Lp_s output; Lr_s output; deu_dap input; DCLw input; Yv_n input; Nv_n input; qbar input; D input; Nv_ns output
function [Yv_ns,Lv_s,Lp_s,Lr_s,Nv_ns] = Get_YLNslip(b,Xp_dash,xp,yp,Xp,deu_dap,DCLw,Yv_n,Nv_n,qbar,D)
% This block estimates the slipstream effect on lateral and directional
% aeroderivatves using NASA TN D-6946

% written by A Cooke 24 Jan 08

Del_qbar_ratio = (4 * Xp)/(qbar * pi * D^2);
slip_factor    = Del_qbar_ratio - deu_dap*(1 + Del_qbar_ratio);

Yv_ns = Yv_n * slip_factor;
Nv_ns = Nv_n * slip_factor;
Lv_s  = 0.5 * (Xp_dash/b) * DCLw * (1 - deu_dap);
Lp_s  = -4 * DCLw * (yp/b)^2;
Lr_s  =  2 * DCLw * (xp/b)^2;

== matlab function AssembledTEST1/Subsystem/Powerplants and Slipstream/Subsystem2/Powerplant - starboard (forces and moments about spinner) (in body axes)/Get_Del_qhq/Embedded MATLAB Function1 ==
  data: ep input; DelMp_q output; eu input; TC input; Iwn2 input
function DelMp_q = getDelMp(ep,eu,TC,Iwn2)
% This block determines the change in free moments for the
% nacelle due to slipstream effects, see NASA TN D-6800

% Author: A Cooke - 26 Oct 07

Del_qw_q = TC * 8/pi;
DelMp_q = (180/pi)*(eu - ep)*(1 + Del_qw_q)*Iwn2/36.5;

== matlab function AssembledTEST1/Subsystem/Powerplants and Slipstream/Subsystem2/Powerplant - starboard (forces and moments about spinner) (in body axes)/Propeller - right (forces and moments about spinner) (in body axes)/Embedded MATLAB Function ==
  data: CT input; beta0 input; sigma_e input; CZ_alpha output; CN_alpha output; J input
function [CZ_alpha,CN_alpha] = PropDevs(CT,beta0,sigma_e,J)

% This function determines the propeller derivatives
% at the specified Power Coefficient and Advance Ratio
%
% Author: A Cooke Date: 7 Jun 06, modified 26 Oct 06

Tc = CT * 8/(pi * J^2);
kb = tan(d2r(beta0 - 5))/(sigma_e * cos(d2r(beta0 - 5)));
CZ_alpha = -((4.25 * sigma_e)/(1 + 2 * sigma_e)) * sin(d2r(beta0 + 3)) * (1 + ((3 * Tc/8)/sqrt(1 + (2*Tc/3))));
CZ_alpha = CZ_alpha * (CT/Tc);
CN_CZ    = -(0.321/(sigma_e + tan(d2r(beta0 + 5)))) * (1 + ((Tc * kb/3)/(1 + (3 * Tc * sqrt(kb)/4))));
CN_alpha = CN_CZ * CZ_alpha;

function rad = d2r(deg)

%   This function converts degrees to radians
%
%   Author: A Cooke Date: 5 May 2004

rad = deg * pi/180;

== matlab function AssembledTEST1/Equations of Motion/Rotational_Kinematic_Transform ==
  data: angles input; rates input; anglesDot output
function anglesDot   = rotationalkinematic(angles, rates)

phi = angles(1);
theta = angles(2);

P = rates(1);
Q = rates(2);
R = rates(3);

transfMat = [1, sin(phi).*tan(theta), cos(phi).*tan(theta);...
			0, cos(phi), -sin(phi);...
			0, sin(phi).*sec(theta), cos(phi).*sec(theta)];

anglesDot = transfMat*[P; Q; R];

end

== matlab function AssembledTEST1/Gravitational_Forces_Moments ==
  data: angles input; d input; mass input; Fg output; Mg output
function [Fg, Mg] = gravityFn(angles, d, mass)

dx = d(1);
dy = d(2);
dz = d(3);

phi = angles(1);
theta = angles(2);

gMat = [-mass*9.81*sin(theta);
		mass*9.81*sin(phi)*cos(theta);
		mass*9.81*cos(phi)*cos(theta)];

mat = [1, 0, 0;
		0, 1, 0;
		0, 0, 1;
		0, -dz, dy;
		dz, 0, -dx; % it is wrong in the notes, there, the terms are swapped and dx does not have the "minus sign"
		-dy, dx, 0];
    
X = mat*gMat;

Fg = [X(1); X(2); X(3)];
Mg = [X(4); X(5); X(6)];
end
